simulink model "10_Zener_Voltage_Regulator"  (R2014a)
settings: Solver=ode23tb  StartTime=0.0  StopTime=.06  RelTol=1e-6
libraries: powerlib x18, simulink x1
settings Model: Creator=CHANDRA BABU  LastModifiedBy=Divya M
settings SolverCC: ZeroCrossControl=DisableAll
settings DataIOCC: SignalLoggingSaveFormat=ModelDataLogs
settings OptimizationCC: ExpressionDepthLimit=2147483647
settings DebuggingCC: UnderspecifiedInitializationDetection=Classic  FcnCallInpInsideContextMsg=UseLocalSettings  StateNameClashWarn=warning
settings GRTTargetCC: CombineOutputUpdateFcns=off  GRTInterface=on

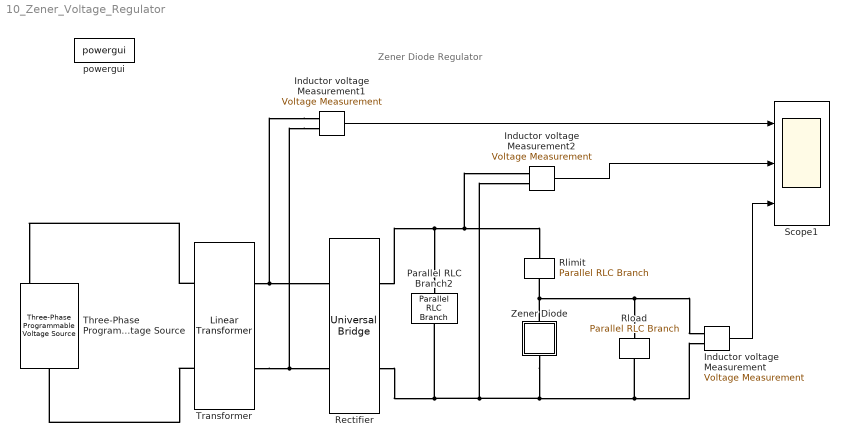
== system 10_Zener_Voltage_Regulator ==
  note: Zener Diode Regulator
  Inductor voltage Measurement : powerlib/Measurements/Voltage Measurement  PhasorSimulation=off  OutputType=Magnitude  PSBequivalent=0
  Inductor voltage Measurement1 : powerlib/Measurements/Voltage Measurement  PhasorSimulation=off  OutputType=Magnitude  PSBequivalent=0
  Inductor voltage Measurement2 : powerlib/Measurements/Voltage Measurement  PhasorSimulation=off  OutputType=Magnitude  PSBequivalent=0
  Parallel RLC Branch2 : powerlib/Elements/Parallel RLC Branch  LConnTagsString=a  RConnTagsString=__new0  BranchType=C  Resistance=200  Inductance=1.0  SetiL0=off  InitialCurrent=0  Capacitance=1e-3  Setx0=off  InitialVoltage=0  Measurements=None
  Rectifier : powerlib/Power Electronics/Universal Bridge  Arms=2  SnubberResistance=1e3  SnubberCapacitance=1e-7  Device=Diodes  Ron=1e-3  Lon=0  ForwardVoltages="[  0  0  ]"  ForwardVoltage=0  GTOparameters=[ 10e-6 , 20e-6 ]  IGBTparameters=[ 1e-6 , 2e-6 ]  Measurements=None  Measurements_2=None  converterType=Rectifier
  Rlimit : powerlib/Elements/Parallel RLC Branch  LConnTagsString=a  RConnTagsString=__new0  BranchType=R  Resistance=40  Inductance=1.0  SetiL0=off  InitialCurrent=0  Capacitance=1e-5  Setx0=off  InitialVoltage=0  Measurements=None
  Rload : powerlib/Elements/Parallel RLC Branch  LConnTagsString=a  RConnTagsString=__new0  BranchType=R  Resistance=100  Inductance=1.0  SetiL0=off  InitialCurrent=0  Capacitance=1e-5  Setx0=off  InitialVoltage=0  Measurements=None
  Scope1 : Scope  NumInputPorts=3
      settings: YMin=-20~0~0  YMax=20~25~15  SaveName=ScopeData2
  Three-Phase Programmable Voltage Source : powerlib/Electrical Sources/Three-Phase Programmable Voltage Source  PositiveSequence="[120  0 60]"  VariationEntity=Amplitude  VariationType=Ramp  VariationTypeAlt=Step  VariationStep=0.5  VariationRate=50  VariationMagnitude=0.3  VariationFrequency=2  VariationTiming=[0.1 0.2]  VariationPhaseA=off  Amplitudes=[1 0.8 1.2 1.0]  TimeValues=[0 0.1 0.15 0.2]  HarmonicGeneration=off  HarmonicA=[3 0.2 -25 0]  HarmonicB=[2 0.15 35 2]  Timing="[0.05  3]"  BusType=swing  Pref=0  Qref=0  Qmin=-inf  Qmax=inf
  Transformer : powerlib/Elements/Linear Transformer  UNITS=pu  NominalPower=[ 1e3 60 ]  winding1="[ 120  0.002  0.001 ]"  winding2="[ 24  0.002  0.001 ]"  ThreeWindings=off  winding3=[ 315e3 0.002 0.08 ]  RmLm=[ 500 500 ]  Measurements=None  DataType=off
  Zener Diode : Subsystem  mask(Zener Diode){Vz=10, Rzt=10, Rzk=400, Izm=400e-3, Vf=0.7, Ron=1e-3}
      mask prompts: Vz "Zener Voltage Vz (V)"; Rzt "Dynamic Impedance Zzt (ohms)"; Rzk "Knee Impedance Zzk (ohms)"; Izm "Maximum Continuous Current Izm (A)"; Vf "Forward Voltage Drop Vf (V)"; Ron "On Resistance Ron (ohms)"
      mask help:
      | Implements a zener diode block.
      | Use values from standard datasheets to populate block dialog
  powergui : powerlib/powergui  Priority=1  SimulationMode=Discrete  SolverType=Tustin  SampleTime=50e-6  frequency=60  SPID=off  DisableSnubberDevices=off  DisableRonSwitches=off  DisableVfSwitches=off  SwTol=0  Interpol=off  DisplayEquations=off  Ts=0  methode=off  frequencyindice=0  Pbase=100e6  ErrMax=1e-4  Iterations=50  UnitsV=kV  UnitsW=MW  FunctionMessages=off  echomessages=off  HookPort=off  EnableUseOfTLC=off  x0status=blocks  RestoreLinks=warning  ResistiveCurrentMeasurement=off  Frange=[0:2:500]  Ylog=off  Xlog=on  ShowGrid=off  save=off  variable=ZData  structure=0  ZoomFFT=on  StartTime=0.0  cycles=1  DisplayStyle=1  fundamental=60  FreqAxis=off  MaxFrequency=1000  frequencyindicesteady=1  RmsSteady=1  display=off
  wires:
  Inductor voltage Measurement1/1 -> Scope1/1
  Inductor voltage Measurement2/1 -> Scope1/2
  Inductor voltage Measurement/1 -> Scope1/3
  connections:
  Inductor voltage Measurement1/LConn1 -- Transformer/RConn1 -- Rectifier/LConn1
  Inductor voltage Measurement1/LConn2 -- Transformer/RConn2 -- Rectifier/LConn2
  Parallel RLC Branch2/LConn1 -- Rlimit/LConn1 -- Inductor voltage Measurement2/LConn1 -- Rectifier/RConn1
  Inductor voltage Measurement/LConn2 -- Rload/RConn1 -- Rectifier/RConn2 -- Parallel RLC Branch2/RConn1 -- Inductor voltage Measurement2/LConn2 -- Zener Diode/RConn1
  Rlimit/RConn1 -- Rload/LConn1 -- Inductor voltage Measurement/LConn1 -- Zener Diode/LConn1
  Transformer/LConn1 -- Three-Phase Programmable Voltage Source/RConn1
  Transformer/LConn2 -- Three-Phase Programmable Voltage Source/LConn1

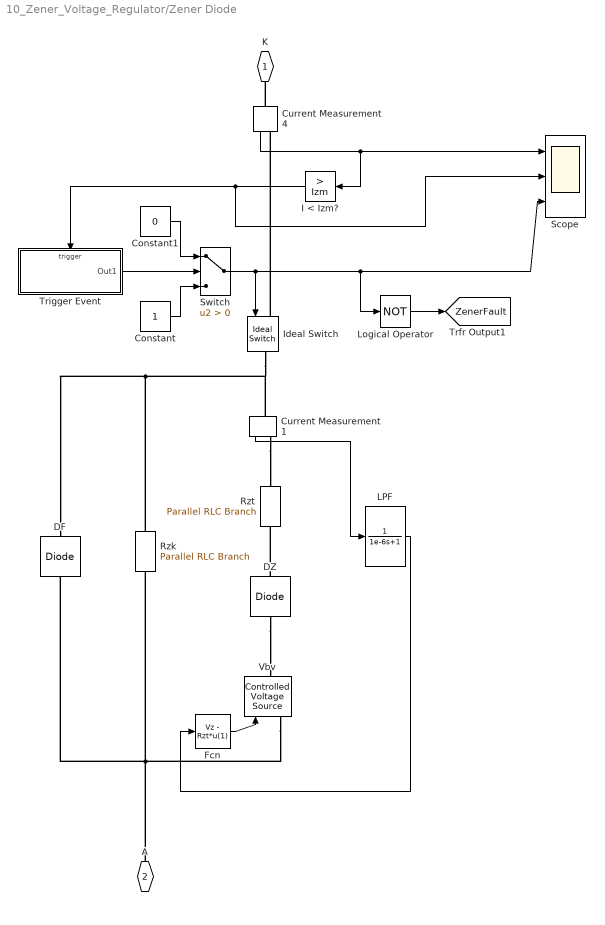
== system 10_Zener_Voltage_Regulator/Zener Diode ==
  Constant : Constant
  Constant1 : Constant  Value=0
  Current Measurement1 : powerlib/Measurements/Current Measurement  PhasorSimulation=off  OutputType=Complex  PSBequivalent=0
  Current Measurement4 : powerlib/Measurements/Current Measurement  PhasorSimulation=off  OutputType=Complex  PSBequivalent=0
  DF : powerlib/Power Electronics/Diode  Ron=Ron  Lon=0  Vf=Vf  IC=0  UseSnubber=off  Rs=1000  Cs=0  Measurements=off
  DZ : powerlib/Power Electronics/Diode  Ron=1e-6  Lon=0  Vf=0  IC=0  UseSnubber=off  Rs=100  Cs=inf  Measurements=off
  Fcn : Fcn  Expr=Vz - Rzt*u(1)
  I < Izm? : simulink/Logic and Bit Operations/Compare To Constant  relop=>  const=Izm  OutDataTypeStr=boolean
  Ideal Switch : powerlib/Power Electronics/Ideal Switch  Ron=0.001  Lon=0  IC=1  Rs=1e5  Cs=0  Measurements=off
  LPF : TransferFcn  Denominator=[1e-6 1]
  Logical Operator : Logic  Operator=NOT  AllPortsSameDT=off  OutDataTypeStr=boolean
  Rzk : powerlib/Elements/Parallel RLC Branch  LConnTagsString=a  RConnTagsString=__new0  BranchType=R  Resistance=Rzk  Inductance=1.0  SetiL0=off  InitialCurrent=0  Capacitance=1e-5  Setx0=off  InitialVoltage=0  Measurements=None
  Rzt : powerlib/Elements/Parallel RLC Branch  LConnTagsString=a  RConnTagsString=__new0  BranchType=R  Resistance=Rzt  Inductance=1.0  SetiL0=off  InitialCurrent=0  Capacitance=1e-5  Setx0=off  InitialVoltage=0  Measurements=None
  Scope : Scope  NumInputPorts=3
      settings: YMin=-2.77556e-017~-1~0.95  YMax=0.4~1~1.05  SaveName=ScopeData4
  Switch : Switch  Criteria=u2 > Threshold
  Trigger Event : Subsystem  TreatAsAtomicUnit=on
  Vbv : powerlib/Electrical Sources/Controlled Voltage Source  Initialize=off  Source_Type=DC  Amplitude=0  Phase=0  Frequency=0  Measurements=None
  K : PMIOPort  Port=1  Side=Left
  A : PMIOPort  Port=2  Side=Right
  tag scope: ZenerFault=global
  wires:
  Fcn/1 -> Vbv/1
  Current Measurement4/1 -> Scope/1, I < Izm?/1
  Current Measurement1/1 -> LPF/1
  LPF/1 -> Fcn/1
  I < Izm?/1 -> Scope/2, Trigger Event/Trigger
  Switch/1 -> Ideal Switch/1, Scope/3, Logical Operator/1
  Trigger Event/1(Out1) -> Switch/2
  Constant/1 -> Switch/3
  Constant1/1 -> Switch/1
  Logical Operator/1 -> [ZenerFault]
  connections:
  DZ/RConn1 -- Vbv/RConn1
  Current Measurement4/LConn1 -- K/RConn1
  DZ/LConn1 -- Rzt/LConn1
  Current Measurement1/RConn1 -- Rzt/RConn1
  Rzk/RConn1 -- Current Measurement1/LConn1 -- Ideal Switch/RConn1 -- DF/RConn1
  Ideal Switch/LConn1 -- Current Measurement4/RConn1
  A/RConn1 -- DF/LConn1 -- Rzk/LConn1 -- Vbv/LConn1

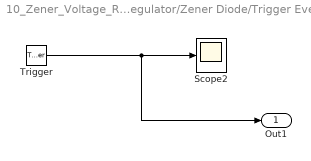
== system 10_Zener_Voltage_Regulator/Zener Diode/Trigger Event ==
  Trigger : TriggerPort  ShowOutputPort=on
  Scope2 : Scope
      settings: YMin=-1  YMax=1
  Out1 : Outport
  wires:
  Trigger/1 -> Scope2/1, Out1/1
